simulink model "flightControlSystem"  (R2021a)
settings: Solver=ode3  StartTime=0  StopTime=TFinal  FixedStep=Ts  RelTol=1e-3  EnableMultiTasking=on
undefined symbols (not defined in the file): BINARIZATION_THRESHOLD, CENTER_THRESHOLD, codertarget, COG_X, COG_Y, Controller, DELAY_LANDING, DERIVATIVE_GAIN, DiscIntNeverNeededParam, Discrete, DISK_KERNEL, Estimator, FLAG_WAIT_FOR_HOVERING, FRAME_SIZE_HEIGHT, FRAME_SIZE_WIDTH, g, G_B_GAIN, GAIN_LANDING, GAIN_TRACK, init, Sensors, strel, Time, TIME_HOLD, Ts, var_acc_angle_N, var_bias_gyr_N, var_gyro_p_N, Vehicle, Z_HIGH, Z_LOW
libraries: simulink x40, pid_lib x4, ctrlSharedLib x4, sharedtransform x3, visionmorphops x1, parrotlib x1
(part 3 of 3)

== matlab function flightControlSystem/Control System/Path Planning/Non linear Path Planner/Y_PLANNER/y_derivative_contribute /derivative error ==
  data: dev_contribute_prev input; derivative_error input; flag_change_error input; dev_contribute output; count_prev input; count output; flag_count_prev input; flag_count output; Ts parameter; TIME_HOLD parameter; DERIVATIVE_GAIN parameter
function [dev_contribute, count, flag_count] = derivative_error(dev_contribute_prev, ...
    derivative_error, flag_change_error,count_prev,flag_count_prev, Ts, ...
    TIME_HOLD, DERIVATIVE_GAIN)
% This MATLAB function computes the derivative contribution of the path planner
% for the x coordinate.
%
% Inputs:
% - dev_contribute_prev: previous value derative part of the planner
% - derivative_error: derivative error value.
% - flag_change_error: it is raised when the sign of the error changes
% - count_prev: previous value of the counter. 
%
% Parameters:
% - Ts: sampling Time.
% - TIME_HOLD: time to which the previous value assumed by the derivative
% contribute has to be hold.
% - DERIVATIVE_GAIN: gain used for the derivative contribution.
%
% Output:
% - dev_contribute: derivative contribution of the path planner.
% - count: counter value
% - flag_count: flag raises when the derivate contribute does not more take
% part to the pat planner.

persistent count_to_be_hold

if isempty(count_to_be_hold)
    count_to_be_hold = round(TIME_HOLD/Ts);
end

flag_count = 0;

if flag_change_error && count_prev == 0    
    flag_count=1;   
end
   
if flag_count_prev || flag_count
    
    if count_prev == count_to_be_hold

        count=0;
        flag_count=0;

    else

        count=count_prev+1;
        flag_count=1;
        
    end
    
    dev_contribute=derivative_error*DERIVATIVE_GAIN;
    
    if dev_contribute ==0 && dev_contribute_prev ~=0 
        
        dev_contribute=dev_contribute_prev;
        
    end

else
    
    flag_count = 0;
    count = 0;
    dev_contribute = 0;
    
end

== stateflow chart flightControlSystem/Control System/Path Planning/Non linear Path Planner/Y_PLANNER/y_linear_contribute ==
  state STATE [group]
    - TRACKING: the drone is tracking the lane or the end-marker.
    - LANDING: the drone lands when the end-marker is detected and the error between the drone CoG and the middle
    of the end-marker is less than MAX_ERROR_LANDING.
    - TRACK_DETECTED: the Image Processing System detected the lane.
    - END_MARKER_DETECTED: the Image Processing System detected the end-marker.
  state INPUT [group]
    - flag_track: flag raised when the lane is detected by Image Processing System.
    - flag_end_marker_to_controller: flag raised when the drone has to land.
    - lin_part: linear part of the path planner.
    - dev_part: derivative part of the path planner.
    - y_estimated: y coordinate of the drone position.
    - flag_end_marker: flag raised when the end-marker is detected by Image Processing System.
  state PARAMETERS [group]
    - GAIN_TRACK: gain used by the drone reference generator to follow the lane.
    - GAIN_LANDING: gain used by the drone reference generator to land over the end-marker.
  state OUTPUT [group]
    - y_planned: y coordinate of the goal position.
  state END_MARKER_DETECTED
    during:
    linear_part = error * GAIN_LANDING;
  state IDLE
  state TRACK_DETECTED
    during:
    linear_part = error * GAIN_TRACK;
  TRACK_DETECTED -> END_MARKER_DETECTED : [flag_end_marker==1 && flag_track==0]
  IDLE -> TRACK_DETECTED : [flag_end_marker==1 && flag_track==0]
  (default) -> IDLE
  data: error input double; GAIN_TRACK parameter double; GAIN_LANDING parameter double; flag_end_marker input double; flag_track input double; linear_part output double

== stateflow chart flightControlSystem/Control System/Path Planning/Non linear Path Planner/Z PLANNER/Chart ==
  state STATE [group]
    - TRACKING: The drone is tracking the lane or the end-marker when they are detected.
    - LANDING: The drone is landing when the land-marker is detected and the error between the drone CoG and
    the central point of the end-marker is less than MAX_ERROR_LANDING.
  state INPUT [group]
    - flag_track: flag raised when the lane is detected by the Image Processing System.
    - flag_end_marker: flag raised when the end-marker is detected by the Image Processing System.
    - norm error: error between the drone CoG and the central point of the end-marker.
  state OUTPUT [group]
    - z_planned: drone altitude sent to the drone controller.
    - flag_end_marker_to_controller: flag raise when the drone has to land.
  state TRACKING
    entry:
    z_planned =  -0.7  ;
    flag_end_marker_to_controller=0;
  state LANDING
    entry:
    z_planned =  0.2 ;
    flag_end_marker_to_controller=1;
  state IDLE
    entry:
    z_planned =  -0.7 ;
    flag_end_marker_to_controller=0;
  (default) -> IDLE
  IDLE -> TRACKING : [after(10,sec)]
  TRACKING -> LANDING : [flag_end_marker==1 && norm_error <= MAX_ERROR_LANDING]
  data: norm_error input double; z_planned output double; MAX_ERROR_LANDING parameter double; flag_end_marker input; flag_track input; flag_end_marker_to_controller output double

== matlab function flightControlSystem/Control System/Path Planning/Non linear Path Planner/Z PLANNER/MATLAB Function ==
  data: norm_error_tot output; error_x input; norm_error output; error_y input; flag_end_marker input; norm_error_prev input
function [norm_error_tot, norm_error] = error_function(error_x, error_y, ...
flag_end_marker, norm_error_prev)
% This MATLAB function computes the norm of the error between the drone CoG
% drone and the middle of point of the end-marker. The norm error is
% computed only if the end-marker is detected.
%
%
%Inputs:
% - error_x: error along the x-axis between the drone CoG and the central 
% point of the end-marker.
% - error_y: error along the y-axis between the drone CoG and the central 
% point of the end-marker.
% - flag_end_marker: the flag indicates when the end-marker is detected.
% - norm_error_prev: previous value of the norm of the error.                                                                                                                                              
%  
%
%Outputs:
% - norm_error_tot: norm of the error between the drone CoG and the central 
% point of the end-marker. It consideres the previous value assumed by the
% norm of the error. The values is condisdered  at the time k = time_step +
% DELAY_LANDING \cdot sampling time. 
% - norm_error: actual value assumed by the norm of error. The error is 
% computed by the drone CoG and the middle point of the end-marker.

if flag_end_marker
    
    norm_error = sqrt((error_x)^2 + (error_y)^2);
    norm_error_tot = norm_error + norm_error_prev  ;
    
else 
    %100 is a constant value greater than MAX_ERROR_LANDING
    norm_error_tot = 100;
    norm_error = 100;
end

== matlab function flightControlSystem/Image Processing System/Image Binarization ==
  data: r input; binarized_frame output; g input; b input; G_B_GAIN parameter; BINARIZATION_THRESHOLD parameter
function binarized_frame = binarizer(r, g, b,G_B_GAIN, BINARIZATION_THRESHOLD)
% The MATLAB function computes a binarized frame starting from a frame 
% expressed in the RGB file format. 
%
% Inputs:
% - r: Red channel frame
% - g: Green channel frame
% - b: Blue channel frame
%
% Output:
% - binarze_frame: the binarized frame
%
% Parameters:
% - G_B_GAIN: used to reduce the amount of green and blue colors inside the frame
% - BINARIZER_THRESHOLD: threshold to detect only the track inside the frame 

frame= r - (g/G_B_GAIN) - (b/G_B_GAIN);

binarized_frame = frame >= BINARIZATION_THRESHOLD;

end

== matlab function flightControlSystem/Control System/Controller/Position Controller/Position error transformation (Earth to Body frame) ==
  data: yaw input; xy_err_earth input; xy_err_body output
function xy_err_body = fcn(yaw,xy_err_earth)

transformation = [cos(yaw), sin(yaw); -sin(yaw),  cos(yaw)];
xy_err_body = transformation * xy_err_earth;


end

== matlab function flightControlSystem/Image Processing System/Red Marker Detection ==
  data: center_x output; center_y output; binary input; error_x_end_marker output; FRAME_SIZE_WIDTH parameter; FRAME_SIZE_HEIGHT parameter; COG_X parameter; COG_Y parameter; CENTER_THRESHOLD parameter; error_y_end_marker output; flag_marker output; flag_grabber_ready output
function [center_x,center_y,error_x_end_marker, error_y_end_marker, flag_marker, ...
    flag_grabber_ready] = red_marker_detector(binary,FRAME_SIZE_WIDTH,... 
FRAME_SIZE_HEIGHT,COG_X, COG_Y, CENTER_THRESHOLD)
% The MATLAB function computes the errors along the x- and y-axis between
% the drone COG and the middle of the lane. The end marker is detected by 
% using a disk kernel. This function is active only when the drone has 
% arrived at the end of the path.
%
%
% Inputs:
% - binary: binarized frame obtained as the convolution with a disk kernel
%
% Outputs:
% - error_y_end_marker: error between the CoG of the drone and a point of the 
% lane in the forward direction along the y-axis. It is expressed in
% pixels.
% - error_x_end_maker: error between the CoG of the drone and a point of the 
% lane in the forward direction along the x-axis. It is expressed in pixels. 
% - flag_end_marker: it is TURE if the Image Processing System detects 
% the end marker.
% - yaw: heading angle of the lane in the image plane.
%
%
%Parameters:
% - COG_X: position of the drone CoG along x-axis of the reference frame.
% - COG_Y: position of the drone CoG along y-axis of the reference frame.
% - FRAME_SIZE_WIDTH: width of the frame.
% - FRAME_SIZE_HEIGHT: height of the frame.

persistent column_accumulator
persistent count_pixel
persistent row_accumulator




if isempty(column_accumulator)
    column_accumulator = 0;
end

if isempty(count_pixel)
    count_pixel = 0;
end

if isempty(row_accumulator)
    row_accumulator = 0;
end

%accumulate all the circle pixels
for i=1:FRAME_SIZE_HEIGHT

    for j=1:FRAME_SIZE_WIDTH

        %check all the pixel belonging to the end marker
        if binary(i,j)==1
            count_pixel = count_pixel +1;
            column_accumulator = column_accumulator + j;
            row_accumulator = row_accumulator + i;

        end

    end
end

%check if a marker is detected
if count_pixel ~= 0
    flag_marker = 1;
    center_x = round(row_accumulator/count_pixel);
    center_y = round(column_accumulator/count_pixel);
else
    flag_marker=0;
    center_x=1;
    center_y=1;
end


% Calculate the medium point of the end marker
error_x_end_marker = -(center_x - COG_X);
error_y_end_marker = (center_y - COG_Y);

% check if the drone is near the circle center
if flag_marker && (abs(error_x_end_marker) <= CENTER_THRESHOLD)&&...
    (abs(error_y_end_marker) <= CENTER_THRESHOLD)
    flag_grabber_ready = 1;
else 
    flag_grabber_ready = 0;
end

% reset of the persistent variables
column_accumulator = 0;
row_accumulator = 0;
count_pixel = 0;


end

== stateflow chart flightControlSystem/Control System/Path Planning/state flow ==
  state Takeoff
    entry:
    xout = 0.1;
    yout = 0.1;
    zout = -1.1;
  state TrackTarget
    entry:
    zout = -1.1;
    during:
    xout = xplanned;
    yout = yplanned;
    x_planned_stored = xplanned;
    y_planned_stored = yplanned;
  state ApproachEggs
    entry:
    xout = x_planned_stored;
    yout = y_planned_stored;
    zout = -1.1;
  (default) -> Takeoff
  Takeoff -> TrackTarget : [after(3,sec) && flag_hover]
  TrackTarget -> ApproachEggs : [flag_grabber_ready]
  data: flag_grabber_ready input; xplanned input; yplanned input; xout output single; yout output single; zout output single; flag_hover input; x_planned_stored local; y_planned_stored local

== stateflow chart flightControlSystem/Control System/Path Planning/Non linear Path Planner/X_PLANNER/Chart1 ==
  state STATE [group]
    - TRACKING: The drone is tracking the lane or the end-marker.
    - LANDING: The drone is landing if the end-marker is detected and the error between the drone CoG and the middle
    point of the end-marker is less than MAX_ERROR_LANDING.
    - TRACK_DETECTED: The Image Processing System detected the lane.
    - END_MARKER_DETECTED: The Image Processing System detected the end-marker.
  state INPUT [group]
    - flag_track: flag raised when the track is detected by the Image Processing System.
    - flag_end_marker_to_controller: flag raised when the drone has to land.
    - lin_part: linear part of the path planner.
    - dev_part: derivative part of the path planner.
    - x_estimated: postion x estimated from the sensors.
    - flag_end_marker: flag raised when the land-marker is detected by the Image Processing System.
  state OUTPUT [group]
    - x_planned: x coordinate of the goal position.
  state TRACKING
    state TRACK_DETECTED
      during:
      x_planned = x_estimated + lin_part + dev_part;
      x_planned_stored = x_planned;
    state END_MARKER_DETECTED
      during:
      x_planned = x_estimated + lin_part ;
      x_planned_stored = x_planned;
    (default) -> TRACK_DETECTED
    TRACK_DETECTED -> END_MARKER_DETECTED : [flag_end_marker==1 && flag_track==0]
    END_MARKER_DETECTED -> TRACK_DETECTED : [flag_end_marker==0 && flag_track==1]
  state LANDING
    during:
    x_planned=x_planned_stored;
  state IDLE
    x_planned=0;
  note: [after(10,sec)]
  (default) -> IDLE
  IDLE -> TRACKING
  TRACKING -> LANDING : [flag_end_marker_to_controller==1]
  data: dev_part input double; lin_part input double; x_planned output double; flag_end_marker_to_controller input double; x_estimated input double; flag_track input double; x_planned_stored local double; flag_end_marker input double
